simulink model "main"  (R2022b)
settings: Solver=FixedStepDiscrete  StartTime=0.0  StopTime=10.0  FixedStep=0.1  RelTol=1e-3  EnableMultiTasking=on
settings Model: TunableVars=PWMA_tl,PWMA_tr,PWMB_tl,PWMB_tr,x,y  TunableVarsStorageClass=Auto,Auto,Auto,Auto,Auto,Auto  TunableVarsTypeQualifier=,,,,,  Creator=TestUser  LastModifiedBy=kylecombest
settings SolverCC: AlgebraicLoopSolver=TrustRegion  AutoInsertRateTranBlk=on
settings DataIOCC: LimitDataPoints=on  ReturnWorkspaceOutputs=off
settings OptimizationCC: EnhancedBackFolding=on  PassReuseOutputArgsAs=Individual arguments  ZeroExternalMemoryAtStartup=off  ZeroInternalMemoryAtStartup=off  OptimizeBlockOrder=speed  DifferentSizesBufferReuse=on  OptimizationCustomize=off  EfficientTunableParamExpr=on
settings DebuggingCC: ParameterTunabilityLossMsg=error  UnconnectedInputMsg=warning  UnconnectedOutputMsg=warning  UnconnectedLineMsg=warning  AllowSymbolicDim=off  SFUnexpectedBacktrackingDiag=warning  SFNoUnconditionalDefaultTransitionDiag=warning  SFExecutionAtInitializationDiag=none  ArithmeticOperatorsInVariantConditions=warning
settings ModelReferenceCC: EnableRefExpFcnMdlSchedulingChecks=on
settings SFSimCC: SimUseLocalCustomCode=off  MATLABDynamicMemAlloc=off  CustomCodeUndefinedFunction=UseInterfaceOnly
settings RTWCC: Description=Embedded Coder  SystemTargetFile=ert.tlc  GenCodeOnly=on  TemplateMakefile=ert_default_tmf  RTWUseLocalCustomCode=off  DLArmComputeVersion=19.05
settings CodeAppCC: ForceParamTrailComments=on  IgnoreCustomStorageClasses=off  OperatorAnnotations=on  SimulinkDataObjDesc=on  SFDataObjDesc=on  InsertBlockDesc=on
settings ERTTargetCC: GenerateSampleERTMain=on  ERTCustomFileTemplate=example_file_process.tlc
settings ConfigComp: CovMetricSettings=dw  CovSaveCumulativeToWorkspaceVar=on  CovSaveSingleToWorkspaceVar=on  CovExternalEMLEnable=off  CovSFcnEnable=off

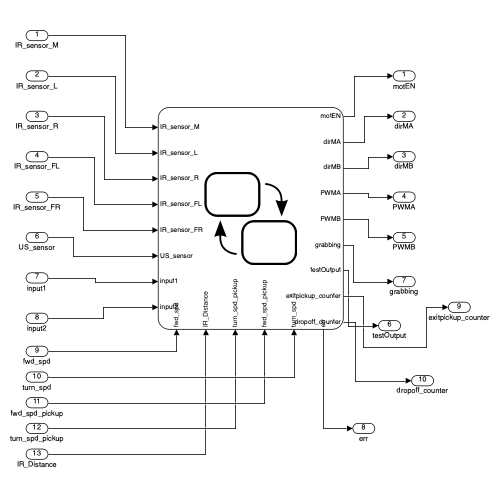
[thumbnail: Simulink's stored preview of the top-level diagram]
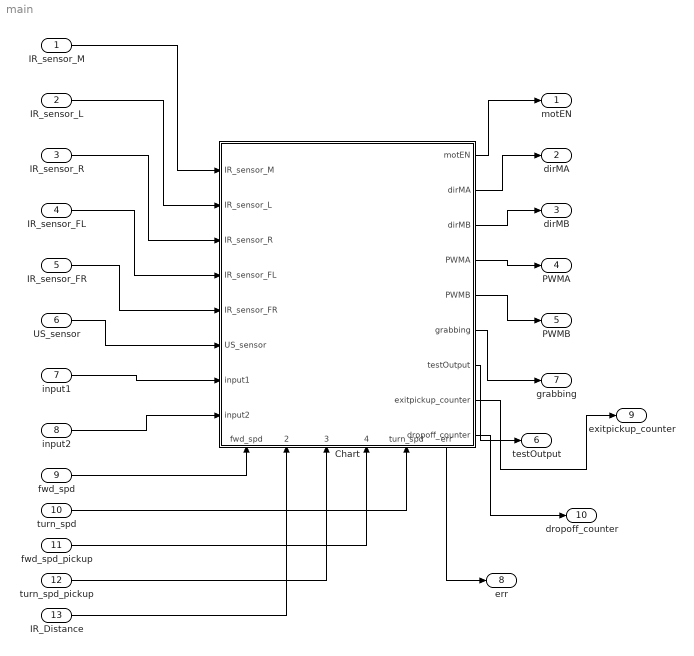
== system main ==
  IR_sensor_M : Inport
  IR_sensor_L : Inport  Port=2
  IR_sensor_R : Inport  Port=3
  IR_sensor_FL : Inport  Port=4
  IR_sensor_FR : Inport  Port=5
  US_sensor : Inport  Port=6
  input1 : Inport  Port=7
  input2 : Inport  Port=8
  fwd_spd : Inport  Port=9
  turn_spd : Inport  Port=10
  fwd_spd_pickup : Inport  Port=11
  turn_spd_pickup : Inport  Port=12
  IR_Distance : Inport  Port=13
  Chart : Stateflow chart  TreatAsAtomicUnit=on
      settings: PortSchema="{\"entries\":[{\"content\":{\"sides\":[{\"content\":{\"connectorIds\":[\"In6\",\"In7\",\"In8\",\"In9\",\"In10\",\"In11\",\"In12\",\"In13\"]},\"type\":\"ConnectorPlacement.EquallySpacedRectSide\",\"uuid\":\"43f03211-d86a-43f4-92ba-476705433e91\"},{\"content\":{\"connectorIds\":[\"Out2\",\"Out3\",\"Out4\",\"Out5\",\"Out6\",\"Out7\",\"Out8\",\"Out9\",\"Out10\"],\"side\":\"RIGHT\"},\"type\":\"ConnectorPlacement.EquallySpacedRectSide\",\"uuid\":\"7770db13-7521-4160-b726-afe2088cf3cd\"},{\"content\":{\"connectorIds\":[],\"side\":\"TOP\"},\"type\":\"ConnectorPlacement.EquallySpacedRectSide\",\"uuid\":\"65bf6453-deff-495e-85b4-05a668c78aaf\"},{\"content\":{\"connectorIds\":[\"In1\",\"In2\",\"In3\",\"In4\",\"In5\",\"Out1\"],\"side\":\"BOTTOM\"},\"type\":\"ConnectorPlacement.EquallySpacedRectSide\",\"uuid\":\"4e5d78fb-35b3-4fb4-a49e-1885b1ff5b01\"}]},\"type\":\"ConnectorPlacement.EquallySpacedConnector\",\"uuid\":\"b6a6359e-0876-4a40-a38b-12efa2c34733\"}],\"packageUris\":[\"http://schema.mathworks.com/mf0/Connector/R2020b\"],\"version\":\"1.0\"}"
  motEN : Outport
  dirMA : Outport  Port=2
  dirMB : Outport  Port=3
  PWMA : Outport  Port=4
  PWMB : Outport  Port=5
  testOutput : Outport  Port=6
  grabbing : Outport  Port=7
  err : Outport  Port=8
  exitpickup_counter : Outport  Port=9
  dropoff_counter : Outport  Port=10
  wires:
  IR_sensor_M/1 -> Chart/6(IR_sensor_M)
  IR_sensor_L/1 -> Chart/7(IR_sensor_L)
  IR_sensor_R/1 -> Chart/8(IR_sensor_R)
  IR_sensor_FL/1 -> Chart/9(IR_sensor_FL)
  IR_sensor_FR/1 -> Chart/10(IR_sensor_FR)
  US_sensor/1 -> Chart/11(US_sensor)
  Chart/2(motEN) -> motEN/1
  Chart/3(dirMA) -> dirMA/1
  Chart/4(dirMB) -> dirMB/1
  Chart/5(PWMA) -> PWMA/1
  Chart/6(PWMB) -> PWMB/1
  input1/1 -> Chart/12(input1)
  input2/1 -> Chart/13(input2)
  Chart/8(testOutput) -> testOutput/1
  Chart/7(grabbing) -> grabbing/1
  Chart/1(err) -> err/1
  fwd_spd/1 -> Chart/1(fwd_spd)
  turn_spd/1 -> Chart/5(turn_spd)
  fwd_spd_pickup/1 -> Chart/4(fwd_spd_pickup)
  turn_spd_pickup/1 -> Chart/3(turn_spd_pickup)
  IR_Distance/1 -> Chart/2(IR_Distance)
  Chart/9(exitpickup_counter) -> exitpickup_counter/1
  Chart/10(dropoff_counter) -> dropoff_counter/1

== stateflow chart main/Chart ==
  state HARDLEFT1
    en:
    testOutput = 5;
    du:
    motEN = 1;
    dirMA = 1;
    dirMB = 0;
    PWMA = turn_spd;
    PWMB = turn_spd;
    left_counter = left_counter + 1
  state IDLE
    en:
    testOutput = 0;
    x = 0;
    y = 0;
    grabbing = 0;
    du:
    motEN = 1;
    dirMA = 1;
    dirMB = 1;
    PWMA = 0;
    PWMB = 0;
    exitpickup_counter = 0;
    left_counter = 0;
    dropoff_counter = 0;
    drop_check = 0;
  state HARDRIGHT_DROPOFF
    en:
    testOutput = 20;
    motEN = 1;
    dirMA = 0;
    dirMB = 1;
    PWMA = turn_spd_pickup;
    PWMB = 0.9*turn_spd_pickup;
    drop_check = 1;
    du:
    testOutput = 100;
    motEN = 1;
    dirMA = 0;
    dirMB = 1;
    PWMA = turn_spd_pickup;
    PWMB = 0.9*turn_spd_pickup;
  state HARDLEFT_DROPOFF
    en:
    testOutput = 9;
    motEN = 1;
    dirMA = 1;
    dirMB = 0;
    PWMA = 0.75*turn_spd_pickup;
    PWMB = turn_spd_pickup;
    du:
    testOutput = 100;
    motEN = 1;
    dirMA = 1;
    dirMB = 0;
    PWMA = 0.75*turn_spd_pickup;
    PWMB = turn_spd_pickup
  state FORWARD
    en:
    testOutput = 1;
    du:
    motEN = 1;
    dirMA = 0;
    dirMB = 0;
    err = IR_sensor_L - IR_sensor_R;
    PWMA = fwd_spd+0.3*err;
    PWMB = fwd_spd-0.3*err;
  state DROPOFFZONE
    en:
    dropoff_counter = dropoff_counter + 1;
    testOutput = 19;
    motEN = 1;
    dirMA = 1;
    dirMB = 1;
    PWMA = 0;
    PWMB = 0;
    du:
    testOutput = 100;
    motEN = 1;
    dirMA = 1;
    dirMB = 1;
    PWMA = 0;
    PWMB = 0;
  state STEERLEFT
    en:
    testOutput = 2;
    du:
    motEN = 1;
    dirMA = 1;
    dirMB = 0;
    PWMA = turn_spd;
    PWMB = turn_spd;
  state STEERRIGHT
    en:
    testOutput = 3;
    du:
    motEN = 1;
    dirMA = 0;
    dirMB = 1;
    PWMA = turn_spd;
    PWMB = turn_spd;
  state PAUSE
    en:
    testOutput = 69;
    motEN = 1;
    dirMA = 1;
    dirMB = 1;
    PWMA = 0;
    PWMB = 0;
  state FORWARDDROPOFF
    en:
    testOutput = 15;
    motEN = 1;
    dirMA = 0;
    dirMB = 0;
    PWMA = fwd_spd;
    PWMB = fwd_spd;
  state REVERSE1
    en:
    testOutput = 23;
    du:
    motEN = 1;
    dirMA = 1;
    dirMB = 1;
    PWMA = fwd_spd * 1.05;
    PWMB = fwd_spd*1*05;
  state DROPZONE
    en:
    testOutput = 21;
    motEN = 0;
    dirMA = 1;
    dirMB = 1;
    PWMA = 0;
    PWMB = 0;
  state STOP
    en:
    testOutput = 6;
    du:
    motEN = 1;
    dirMA = 1;
    dirMB = 1;
    PWMA = 0;
    PWMB = 0;
  state HARDLEFT_PICKUP1
    en:
    testOutput = 16;
    motEN = 1;
    dirMA = 1;
    dirMB = 0;
    PWMA = 0.55*turn_spd_pickup;
    PWMB = turn_spd_pickup;
    du:
    testOutput = 100;
    motEN = 1;
    dirMA = 1;
    dirMB = 0;
    PWMA = 0.55*turn_spd_pickup;
    PWMB = turn_spd_pickup
  state PICKUPZONE
    en:
    testOutput = 7;
    motEN = 1;
    dirMA = 1;
    dirMB = 1;
    PWMA = 0;
    PWMB = 0;
    du:
  state HARDRIGHT_PICKUP1
    en:
    testOutput = 17;
    motEN = 1;
    dirMA = 0;
    dirMB = 1;
    PWMA = turn_spd_pickup;
    PWMB = 0.8 * turn_spd_pickup;
    du:
    testOutput = 100;
    motEN = 1;
    dirMA = 0;
    dirMB = 1;
    PWMA = turn_spd_pickup;
    PWMB = 0.8*turn_spd_pickup;
  state FORWARDDELAY1
    en:
    testOutput = 15;
    motEN = 1;
    dirMA = 0;
    dirMB = 0;
    PWMA = fwd_spd_pickup;
    PWMB = fwd_spd_pickup;
  state FORWARDDELAY
    en:
    testOutput = 15;
    motEN = 1;
    dirMA = 0;
    dirMB = 0;
    PWMA = fwd_spd_pickup;
    PWMB = fwd_spd_pickup;
  state PICKUPZONE1
    en:
    testOutput = 7;
    motEN = 1;
    dirMA = 1;
    dirMB = 1;
    PWMA = 0;
    PWMB = 0;
    du:
  state PICKUPZONE2
    en:
    testOutput = 7;
    motEN = 1;
    dirMA = 1;
    dirMB = 1;
    PWMA = 0;
    PWMB = 0;
    du:
  state HARDRIGHT_PICKUP
    en:
    testOutput = 8;
    if exitpickup_counter == 0
    motEN = 1;
    dirMA = 0;
    dirMB = 1;
    PWMA = 0.9*turn_spd_pickup;
    PWMB = turn_spd_pickup;
    elseif exitpickup_counter == 1
    motEN = 1;
    dirMA = 0;
    dirMB = 1;
    PWMA = turn_spd_pickup;
    PWMB = 0.8*turn_spd_pickup;
    else
    motEN = 1;
    dirMA = 0;
    dirMB = 1;
    PWMA = turn_spd_pickup;
    PWMB = 0.8*turn_spd_pickup;
    end
    du:
    testOutput = 100;
    if exitpickup_counter == 0;
    motEN = 1;
    dirMA = 0;
    dirMB = 1;
    PWMA = turn_spd_pickup;
    PWMB = turn_spd_pickup;
    elseif exitpickup_counter == 1
    motEN = 1;
    dirMA = 0;
    dirMB = 1;
    PWMA = turn_spd_pickup;
    PWMB = 0.8*turn_spd_pickup;
    else
    motEN = 1;
    dirMA = 0;
    dirMB = 1;
    PWMA = turn_spd_pickup;
    PWMB = 0.8*turn_spd_pickup;
    end
  state HARDLEFT_PICKUP
    en:
    testOutput = 9;
    if exitpickup_counter == 0;
    motEN = 1;
    dirMA = 1;
    dirMB = 0;
    PWMA = 0.85*turn_spd_pickup;
    PWMB = turn_spd_pickup;
    elseif exitpickup_counter == 1;
    motEN = 1;
    dirMA = 1;
    dirMB = 0;
    PWMA = 0.75*turn_spd_pickup;
    PWMB = turn_spd_pickup;
    else
    motEN = 1;
    dirMA = 1;
    dirMB = 0;
    PWMA = 0.75*turn_spd_pickup;
    PWMB = turn_spd_pickup;
    end
    du:
    testOutput = 100;
    if exitpickup_counter == 0;
    motEN = 1;
    dirMA = 1;
    dirMB = 0;
    PWMA = 0.85*turn_spd_pickup;
    PWMB = turn_spd_pickup;
    elseif exitpickup_counter == 1;
    motEN = 1;
    dirMA = 1;
    dirMB = 0;
    PWMA = 0.75*turn_spd_pickup;
    PWMB = turn_spd_pickup;
    else
    motEN = 1;
    dirMA = 1;
    dirMB = 0;
    PWMA = 0.75*turn_spd_pickup;
    PWMB = turn_spd_pickup;
    end
  state FOWARDDELAY2
    en:
    testOutput = 70;
    motEN = 1;
    dirMA = 0;
    dirMB = 0;
    PWMA = fwd_spd_pickup;
    PWMB = fwd_spd_pickup;
    du:
  state FORWARDDELAY3
    en:
    testOutput = 70;
    motEN = 1;
    dirMA = 0;
    dirMB = 0;
    PWMA = fwd_spd_pickup;
    PWMB = fwd_spd_pickup;
    du:
  state STEERLEFT1
    en:
    testOutput = 11;
    du:
    motEN = 1;
    dirMA = 1;
    dirMB = 0;
    PWMA = 0,9*turn_spd_pickup;
    PWMB = 0.9*turn_spd_pickup;
  state STEERRIGHT1
    en:
    testOutput = 12;
    du:
    motEN = 1;
    dirMA = 0;
    dirMB = 1;
    PWMA = 0.9*turn_spd_pickup;
    PWMB = 0.9*turn_spd_pickup;
  state PICKUPFORWARD
    en:
    testOutput = 10;
    du:
    motEN = 1;
    dirMA = 0;
    dirMB = 0;
    err = IR_sensor_L - IR_sensor_R;
    PWMA = fwd_spd_pickup+0.1*err;
    PWMB = fwd_spd_pickup-0.1*err;
  state STOP_PICKUP
    en:
    grabbing = 1;
    testOutput = 13;
    du:
    motEN = 1;
    dirMA = 1;
    dirMB = 1;
    PWMA = 0;
    PWMB = 0;
  state GRABBING
    en:
    testOutput = 22;
    motEN = 0;
    dirMA = 1;
    dirMB = 1;
    PWMA = 0;
    PWMB = 0;
  state REVERSE
    en:
    testOutput = 14;
    exitpickup_counter = exitpickup_counter + 1
    du:
    motEN = 1;
    dirMA = 1;
    dirMB = 1;
    err = IR_sensor_L - IR_sensor_R;
    PWMA = 1.05*fwd_spd_pickup; %-0.75*err;
    PWMB = 1.05*fwd_spd_pickup; %+0.75*err;
    ;
  state LINEUPREV
    en:
    testOutput = 18;
    du:
    testOutput = 100;
    motEN = 1;
    dirMA = 1;
    dirMB = 1;
    PWMA = 1.05*fwd_spd_pickup;
    PWMB = 1.05*fwd_spd_pickup;
  STEERRIGHT -> HARDLEFT1 [order 2] : [IR_sensor_FL == 0 & IR_sensor_FR == 1 & (left_counter == 0 || exitpickup_counter >= 3)  ]
  (default) -> IDLE
  HARDLEFT1 -> FORWARD : [IR_sensor_R > 750 & IR_sensor_FR == 1 & IR_sensor_FL == 1]
  STEERLEFT -> HARDLEFT1 [order 2] : [IR_sensor_FL == 0 & IR_sensor_FR == 1 & (left_counter == 0 || exitpickup_counter >= 3) ]
  FORWARD -> HARDLEFT1 [order 4] : [IR_sensor_FL == 0 & IR_sensor_FR == 1 & (left_counter == 0 || exitpickup_counter >= 3) ]
  IDLE -> FORWARD : [IR_sensor_M >= 750 & IR_sensor_L >=750 & IR_sensor_L >=750 && IR_sensor_FL == 1 && IR_sensor_FR == 1 & input1 ~=0 & input2~= 0]
  HARDRIGHT_DROPOFF -> FORWARD : [IR_sensor_L > 750 & IR_sensor_FR == 1 & IR_sensor_FL == 1]
  DROPOFFZONE -> HARDRIGHT_DROPOFF [order 1] : [dropoff_counter == input2]
  FORWARD -> DROPOFFZONE [order 6] : [IR_sensor_FR == 0 & exitpickup_counter == 3 & drop_check == 0]
  PAUSE -> HARDLEFT_DROPOFF
  HARDLEFT_DROPOFF -> FORWARD : [IR_sensor_R > 750 & IR_sensor_FR == 1 & IR_sensor_FL == 1]
  FORWARD -> STEERLEFT [order 1] : [IR_sensor_L >= 750 & IR_sensor_R <750 & IR_sensor_M >= 750]
  STEERRIGHT -> FORWARD [order 1] : [IR_sensor_L >= 750 & IR_sensor_R >= 750 & IR_sensor_M >= 750]
  STEERLEFT -> FORWARD [order 1] : [IR_sensor_L >= 750 & IR_sensor_R >= 750 & IR_sensor_M >=750]
  FORWARDDROPOFF -> FORWARD : [IR_sensor_FR == 1]
  STEERRIGHT -> STOP [order 3] : [IR_Distance <825]
  STEERLEFT -> STOP [order 3] : [IR_Distance <825]
  FORWARD -> STEERRIGHT [order 2] : [IR_sensor_L <750 & IR_sensor_R >= 750 & IR_sensor_M >= 750]
  FORWARD -> STOP [order 3] : [IR_Distance <825]
  STEERLEFT -> PICKUPZONE [order 4] : [IR_sensor_FR == 0 && exitpickup_counter == 3 ]
  STOP -> FORWARD [order 1] : [IR_Distance > 825]
  STEERRIGHT -> PICKUPZONE [order 4] : [IR_sensor_FR == 0 && exitpickup_counter < 3 ]
  HARDLEFT_PICKUP1 -> FORWARD : [IR_sensor_R > 750 & IR_sensor_FR == 1 & IR_sensor_FL == 1]
  HARDRIGHT_PICKUP1 -> FORWARD : [IR_sensor_L > 750 & IR_sensor_FR == 1 & IR_sensor_FL == 1]
  PICKUPFORWARD -> FORWARD [order 4] : [exitpickup_counter == 3]
  FORWARD -> PICKUPZONE [order 5] : [IR_sensor_FR == 0 && exitpickup_counter < 3]
  REVERSE1 -> PAUSE : [IR_sensor_FR == 0]
  DROPOFFZONE -> FORWARDDROPOFF [order 2] : [dropoff_counter ~= input2]
  STOP -> DROPZONE [order 2] : [drop_check ==1]
  DROPZONE -> REVERSE1
  FORWARDDELAY -> HARDLEFT_PICKUP1
  PICKUPZONE -> FOWARDDELAY2 [order 4] : [input1 == 2 & exitpickup_counter == 1]
  PICKUPZONE -> FORWARDDELAY3 [order 3] : [input1 == 1 & exitpickup_counter == 1]
  PICKUPZONE -> HARDLEFT_PICKUP [order 1] : [input1 == 1 & (exitpickup_counter == 0 || exitpickup_counter == 2)]
  PICKUPZONE -> HARDRIGHT_PICKUP [order 2] : [input1 == 2 & (exitpickup_counter == 0 || exitpickup_counter == 2)]
  FORWARDDELAY1 -> HARDRIGHT_PICKUP1
  PICKUPZONE1 -> FORWARDDELAY1
  PICKUPZONE2 -> FORWARDDELAY
  REVERSE -> PICKUPZONE1 [order 1] : [IR_sensor_FR == 0 & input1==1]
  REVERSE -> PICKUPZONE2 [order 2] : [IR_sensor_FR == 0 & input1 == 2]
  FOWARDDELAY2 -> HARDRIGHT_PICKUP
  FORWARDDELAY3 -> HARDLEFT_PICKUP
  HARDRIGHT_PICKUP -> PICKUPFORWARD : [IR_sensor_L > 750 & IR_sensor_FR == 1 & IR_sensor_FL == 1]
  HARDLEFT_PICKUP -> PICKUPFORWARD : [IR_sensor_R > 815 & IR_sensor_FR == 1 & IR_sensor_FL == 1]
  STEERRIGHT1 -> PICKUPFORWARD [order 1] : [IR_sensor_L >= 790 & IR_sensor_R >= 790 & IR_sensor_M >= 790]
  STEERLEFT1 -> PICKUPFORWARD [order 1] : [IR_sensor_L >= 790 & IR_sensor_R >= 790 & IR_sensor_M >=790]
  LINEUPREV -> PICKUPFORWARD : [IR_sensor_FL == 0 || IR_sensor_FR == 0]
  PICKUPFORWARD -> STEERRIGHT1 [order 1] : [IR_sensor_L <790 & IR_sensor_R >= 790 & IR_sensor_M >= 790]
  PICKUPFORWARD -> STEERLEFT1 [order 3] : [IR_sensor_L >= 790 & IR_sensor_R <790 & IR_sensor_M >= 790]
  PICKUPFORWARD -> STOP_PICKUP [order 2] : [IR_Distance < 875]
  STEERRIGHT1 -> STOP_PICKUP [order 2] : [IR_Distance < 875]
  STEERLEFT1 -> STOP_PICKUP [order 2] : [IR_Distance < 875]
  STOP_PICKUP -> LINEUPREV [order 2] : [((IR_Distance <900 & (IR_sensor_M < 805 || IR_sensor_R < 780 || IR_sensor_L < 805))) || (IR_sensor_M < 805 & IR_sensor_R < 780 & IR_sensor_L < 805)]
  STOP_PICKUP -> GRABBING [order 1] : [IR_sensor_M > 805 & IR_sensor_R > 780 & IR_sensor_L > 805]
  GRABBING -> REVERSE
  data: fwd_spd input; IR_Distance input; turn_spd_pickup input; fwd_spd_pickup input; turn_spd input; err output; data local; IR_sensor_M input; IR_sensor_L input; IR_sensor_R input; IR_sensor_FL input; IR_sensor_FR input; US_sensor input; motEN output; dirMA output; dirMB output; PWMA output; PWMB output; grabbing output; input1 input; input2 input; PWMB_tr constant double; PWMA_tr constant double; PWMB_tl constant double; PWMA_tl constant double; x local; y local; testOutput output; time local; done local; left_counter local; exitpickup_counter output; dropoff_counter output; drop_check local
